simulink model "teng4_demo2_UDP_slx2py_sender_okclean"  (R2020a)
settings: Solver=FixedStepAuto  StartTime=0.0  StopTime=inf  FixedStep=0.001  RelTol=1e-3
libraries: dspnetwork x1
settings Model: Creator=admin  LastModifiedBy=Teng
settings DataIOCC: ReturnWorkspaceOutputs=off
settings DebuggingCC: ArithmeticOperatorsInVariantConditions=warning
settings SFSimCC: SimUseLocalCustomCode=off  CustomCodeUndefinedFunction=UseInterfaceOnly
settings RTWCC: RTWUseLocalCustomCode=off
settings CodeAppCC: StateflowObjectComments=on

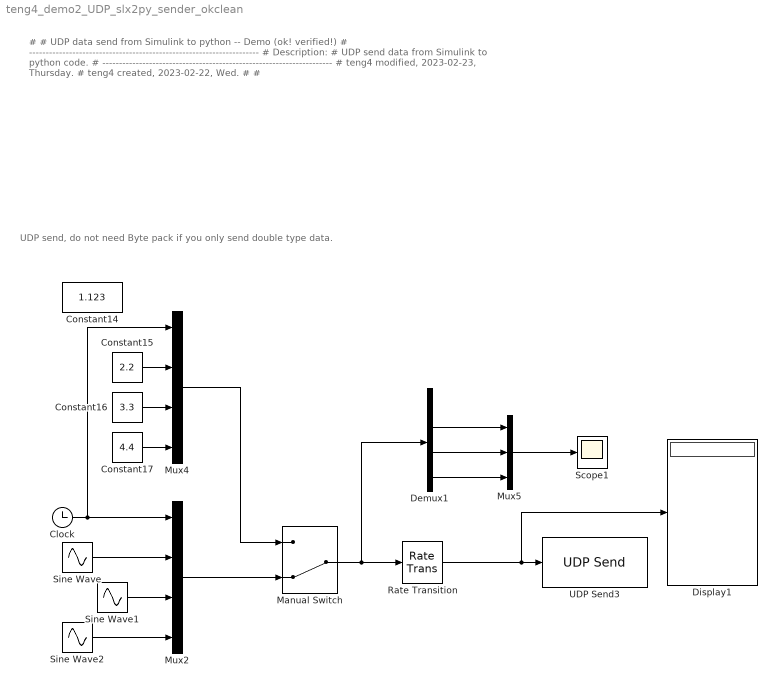
== system teng4_demo2_UDP_slx2py_sender_okclean ==
  note: #
      | # UDP data send from Simulink to python -- Demo (ok! verified!)
      | # ---------------------------------------------------------------------
      | # Description:
      | # UDP send data from Simulink to python code.
      | # ---------------------------------------------------------------------
      | # teng4 modified, 2023-02-23, Thursday.
      | # teng4 created, 2023-02-22, Wed.
      | #
      | #
  note: UDP send,
      | do not need Byte pack if you only send double type data.
  Clock : Clock
  Constant14 : Constant  Value=1.123
  Constant15 : Constant  Value=2.2
  Constant16 : Constant  Value=3.3
  Constant17 : Constant  Value=4.4
  Demux1 : Demux
  Display1 : Display
  Manual Switch : ManualSwitch  CurrentSetting=0
  Mux2 : Mux
  Mux4 : Mux
  Mux5 : Mux  Inputs=3
  Rate Transition : RateTransition  OutPortSampleTime=0.1
  Scope1 : Scope
  Sine Wave : Sin  SampleTime=0
  Sine Wave1 : Sin  Amplitude=0.5  Frequency=2  SampleTime=0
  Sine Wave2 : Sin  Frequency=10  Phase=pi  SampleTime=0
  UDP Send3 : dspnetwork/UDP Send  remoteURL='192.168.1.102'  remotePort=25000  localURL='0.0.0.0'  localPortSource=Automatically determine  localPort=-1  sendBufferSize=8192  sampletime=-1  blockPlatform=[]  separateLengthPort=0
  wires:
  Sine Wave1/1 -> Mux2/3
  Clock/1 -> Mux4/1, Mux2/1
  Sine Wave/1 -> Mux2/2
  Sine Wave2/1 -> Mux2/4
  Mux2/1 -> Manual Switch/2
  Constant15/1 -> Mux4/2
  Constant16/1 -> Mux4/3
  Constant17/1 -> Mux4/4
  Rate Transition/1 -> UDP Send3/1, Display1/1
  Mux4/1 -> Manual Switch/1
  Manual Switch/1 -> Demux1/1, Rate Transition/1
  Mux5/1 -> Scope1/1
  Demux1/3 -> Mux5/2
  Demux1/2 -> Mux5/1
  Demux1/4 -> Mux5/3
